simulink library "servo_hub_lib"  (R2023a)
settings: Solver=VariableStepAuto  StartTime=0.0  StopTime=10.0  RelTol=1e-3
settings Model: Creator=dige  LastModifiedBy=Administrator
settings SolverCC: AlgebraicLoopSolver=TrustRegion
settings OptimizationCC: ReuseModelBlockBuffer=off
settings DebuggingCC: UnconnectedInputMsg=warning  UnconnectedOutputMsg=warning  UnconnectedLineMsg=warning
settings ModelReferenceCC: EnableRefExpFcnMdlSchedulingChecks=on

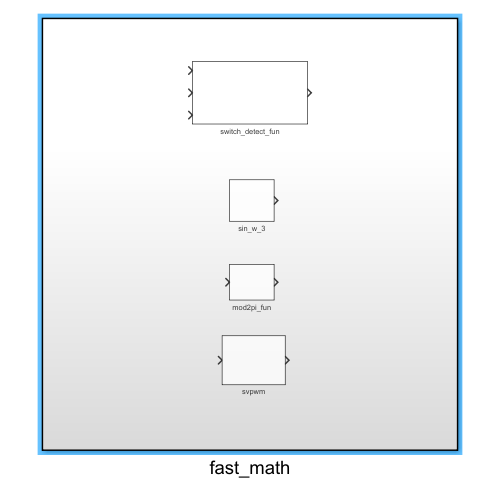
[thumbnail: Simulink's stored preview of the top-level diagram]
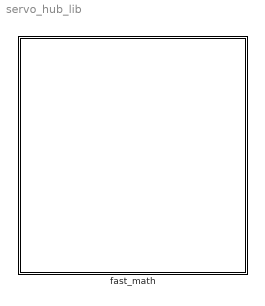
== system servo_hub_lib ==
  fast_math : Subsystem

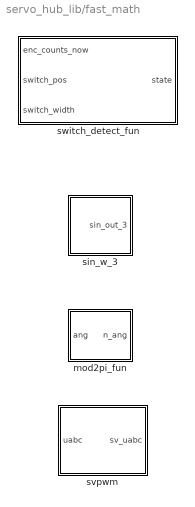
== system servo_hub_lib/fast_math ==
  mod2pi_fun : MATLAB Function  TreatAsAtomicUnit=on
  sin_w_3 : Subsystem  mask{amp=1, frq=1}
      mask prompts: amp "三相正弦赋值"; frq "三相正弦频率"
      mask DialogControl Control1 Prompt: 三相正弦信号发生器，相位各相差120°
  "svpwm " : MATLAB Function
  switch_detect_fun : Subsystem

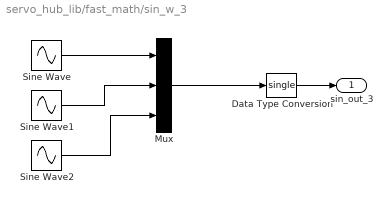
== system servo_hub_lib/fast_math/sin_w_3 ==
  Data Type Conversion : DataTypeConversion  OutDataTypeStr=single  SaturateOnIntegerOverflow=off  RndMeth=Floor
  Mux : Mux  Inputs=3
  Sine Wave : Sin  Amplitude=amp  Frequency=frq
  Sine Wave1 : Sin  Amplitude=amp  Frequency=frq  Phase=2*pi/3
  Sine Wave2 : Sin  Amplitude=amp  Frequency=frq  Phase=-2*pi/3
  sin_out_3 : Outport
  wires:
  Mux/1 -> Data Type Conversion/1
  Data Type Conversion/1 -> sin_out_3/1
  Sine Wave2/1 -> Mux/3
  Sine Wave1/1 -> Mux/2
  Sine Wave/1 -> Mux/1

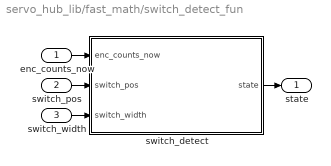
== system servo_hub_lib/fast_math/switch_detect_fun ==
  enc_counts_now : Inport
  switch_pos : Inport  Port=2
  switch_width : Inport  Port=3
  switch_detect : MATLAB Function  TreatAsAtomicUnit=on
  state : Outport
  wires:
  enc_counts_now/1 -> switch_detect/1(enc_counts_now)
  switch_pos/1 -> switch_detect/2(switch_pos)
  switch_detect/1(state) -> state/1
  switch_width/1 -> switch_detect/3(switch_width)

== matlab function servo_hub_lib/fast_math/svpwm  ==
  data: uabc input; sv_uabc output
function sv_uabc  = svpwm_genrate(uabc)
%最大值最小值法
va = single(uabc(1));
vb = single(uabc(2));
vc = single(uabc(3));
sv_uabc = single(zeros(1,3));

if va>vb
    vmax = va;
    vmin = vb;
else
    vmax = vb;
    vmin = va;
end

if vc>vmax
    vmax = vc;
elseif vc<vmin
    vmin = vc;
end

vcom = 0.5*(vmax+vmin);

ua = va-vcom;
ub = vb-vcom;
uc = vc-vcom;

sv_uabc(1) = single(ua);
sv_uabc(2) = single(ub);
sv_uabc(3) = single(uc);

== matlab function servo_hub_lib/fast_math/mod2pi_fun ==
  data: ang input; n_ang output
function n_ang = mod2pi(ang)
    % 将角度限制在0到2π范围内
    TWO_PI = single(2*pi);
    n_ang = single(ang);
    while n_ang < 0
        n_ang = n_ang + TWO_PI;
    end
    while n_ang >= TWO_PI
        n_ang = n_ang - TWO_PI;
    end
end

== matlab function servo_hub_lib/fast_math/switch_detect_fun/switch_detect ==
  data: enc_counts_now input; switch_pos input; state output; switch_width input
function state = switch_detect(enc_counts_now, switch_pos, switch_width)
%% 开关检测函数
% enc_counts_now  编码器当前位置
% switch_pos  开关检测位置
% switch_pos  开关检测宽度 检测宽度中心对称  +- switch_width

if (enc_counts_now <= (switch_pos + switch_width)) ...
&& (enc_counts_now >= (switch_pos - switch_width))
    state = uint8(1);   %触发状态  检测到当前位置处于开关检测区域
else
    state = uint8(0);   %未触发状态  未检测到开关
end
